simulink model "truckParallelParking"  (R2023a)
settings: Solver=VariableStepAuto  StartTime=0.0  StopTime=30  RelTol=1e-3
values from neighbouring files (symbols this model uses):
  Duration = 30    [ParallelParkingOfTruckTrailerUsingMultistageNonlinearMPC1.m]
  initialPose1 = [-15,-30,pi/2,0]'    [ParallelParkingOfTruckTrailerUsingMultistageNonlinearMPC1.m]
  mdlParas = [truckDimensions.M1;truckDimensions.L1;truckDimensions.L2;             truckDimensions.W1;truckDimensions.W2]    [ParallelParkingOfTruckTrailerUsingMultistageNonlinearMPC1.m]
  numParas = numel(mdlParas) + numel(obsParas)    [ParallelParkingOfTruckTrailerUsingMultistageNonlinearMPC1.m]
  obsParas = [wallLength;wallWidth]    [ParallelParkingOfTruckTrailerUsingMultistageNonlinearMPC1.m]
  pPlanning = planner.horizon    [ParallelParkingOfTruckTrailerUsingMultistageNonlinearMPC1.m]    (also in mpcGeneratePlanner.m = 20)
  pTracking = controller.horizon    [ParallelParkingOfTruckTrailerUsingMultistageNonlinearMPC1.m]
  targetPose2 = [-8,-8,pi/2,0]'    [ParallelParkingOfTruckTrailerUsingMultistageNonlinearMPC1.m]
  tmax = tmin + Tsplan    [ParallelParkingOfTruckTrailerUsingMultistageNonlinearMPC1.m]
  tmin = 2.5    [ParallelParkingOfTruckTrailerUsingMultistageNonlinearMPC1.m]
  Ts = controller.sampleTime    [ParallelParkingOfTruckTrailerUsingMultistageNonlinearMPC1.m]    (also in mpcGeneratePlanner.m = 1)
libraries: mpclib x2, simulink x1
settings Model: Creator=The MathWorks, Inc.  LastModifiedBy=The MathWorks, Inc.
settings SolverCC: MaxZcPerStep=1
settings DebuggingCC: UnconnectedInputMsg=warning  UnconnectedOutputMsg=warning  UnconnectedLineMsg=warning
settings ModelReferenceCC: EnableRefExpFcnMdlSchedulingChecks=on
settings RTWCC: DLArmComputeVersion=19.05

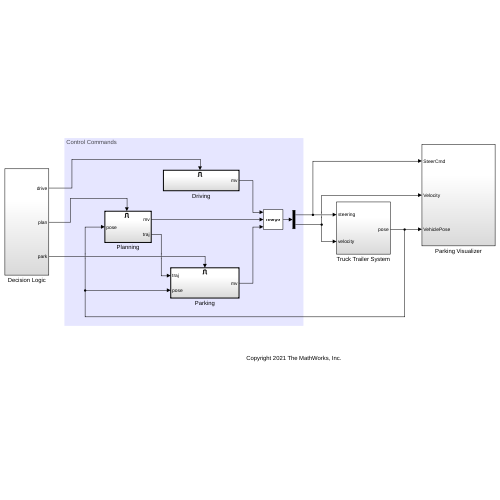
[thumbnail: Simulink's stored preview of the top-level diagram]
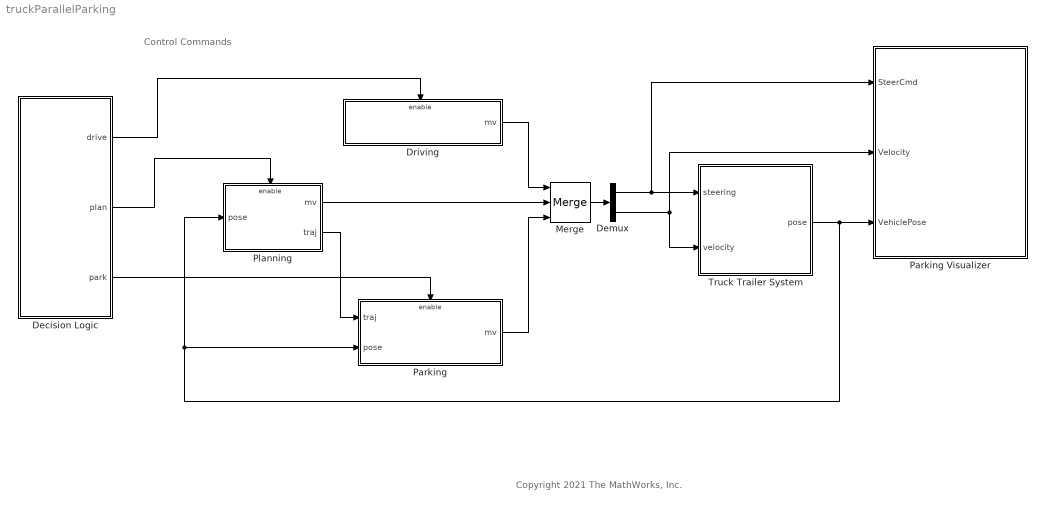
== system truckParallelParking ==
  note: Control Commands
  note: Copyright 2021 The MathWorks, Inc.
  Decision Logic : Subsystem
  Demux : Demux  Outputs=2
  Driving : Subsystem  TreatAsAtomicUnit=on
  Merge : Merge  Inputs=3
  Parking : Subsystem  TreatAsAtomicUnit=on
  Parking Visualizer : Subsystem
  Planning : Subsystem  TreatAsAtomicUnit=on
  Truck Trailer System : Subsystem
  wires:
  Decision Logic/3(park) -> Parking/Enable
  Decision Logic/1(drive) -> Driving/Enable
  Decision Logic/2(plan) -> Planning/Enable
  Merge/1 -> Demux/1
  Driving/1(mv) -> Merge/1
  Demux/1 -> Truck Trailer System/1(steering), Parking Visualizer/1(SteerCmd)
  Demux/2 -> Truck Trailer System/2(velocity), Parking Visualizer/2(Velocity)
  Truck Trailer System/1(pose) -> Parking/2(pose), Planning/1(pose), Parking Visualizer/3(VehiclePose)
  Planning/1(mv) -> Merge/2
  Parking/1(mv) -> Merge/3
  Planning/2(traj) -> Parking/1(traj)

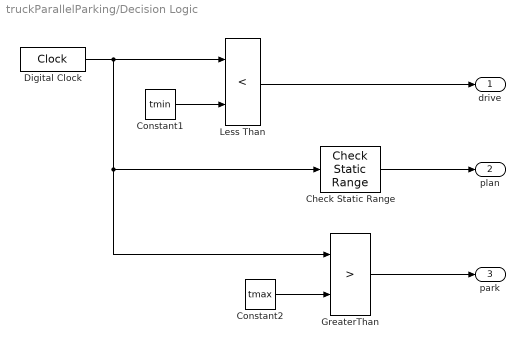
== system truckParallelParking/Decision Logic ==
  Check Static Range : simulink/Model Verification/Check  Static Range  Description=tmin <= u <= tmax  max=tmax  max_included=on  min=tmin  min_included=on  enabled=off  stopWhenAssertionFail=off  export=on  icon=graphic
  Constant1 : Constant  Value=tmin
  Constant2 : Constant  Value=tmax
  Digital Clock : DigitalClock  SampleTime=0.1
  GreaterThan : RelationalOperator  Operator=>  OutDataTypeStr=boolean  RndMeth=Simplest  InputSameDT=off
  Less Than : RelationalOperator  Operator=<  OutDataTypeStr=boolean  RndMeth=Simplest  InputSameDT=off
  drive : Outport
  plan : Outport  Port=2
  park : Outport  Port=3
  wires:
  Constant1/1 -> Less Than/2
  Less Than/1 -> drive/1
  Digital Clock/1 -> GreaterThan/1, Check Static Range/1, Less Than/1
  Check Static Range/1 -> plan/1
  Constant2/1 -> GreaterThan/2
  GreaterThan/1 -> park/1

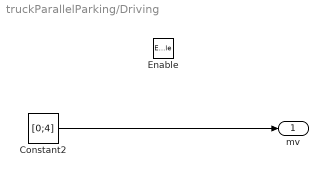
== system truckParallelParking/Driving ==
  Enable : EnablePort  StatesWhenEnabling=reset
  Constant2 : Constant  Value=[0;4]  VectorParams1D=off
  mv : Outport
  wires:
  Constant2/1 -> mv/1

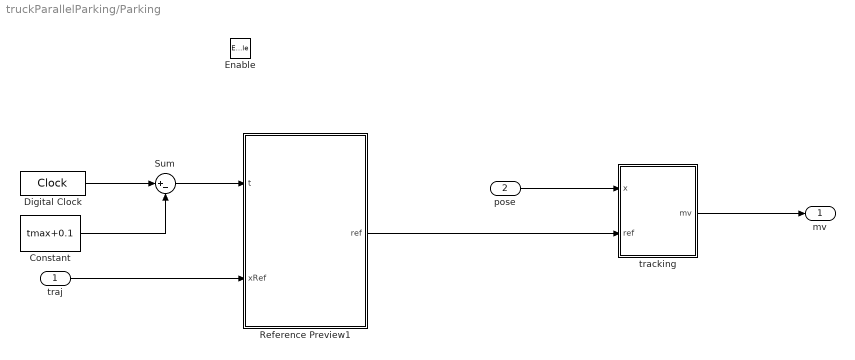
== system truckParallelParking/Parking ==
  traj : Inport
  pose : Inport  Port=2
  Enable : EnablePort  StatesWhenEnabling=reset
  Constant : Constant  Value=tmax+0.1
  Digital Clock : DigitalClock  SampleTime=0.1
  Reference Preview1 : MATLAB Function  TreatAsAtomicUnit=on
  Sum : Sum  Inputs=|+-
  tracking : Subsystem
  mv : Outport
  wires:
  traj/1 -> Reference Preview1/2(xRef)
  Reference Preview1/1(ref) -> tracking/2(ref)
  pose/1 -> tracking/1(x)
  tracking/1(mv) -> mv/1
  Sum/1 -> Reference Preview1/1(t)
  Digital Clock/1 -> Sum/1
  Constant/1 -> Sum/2

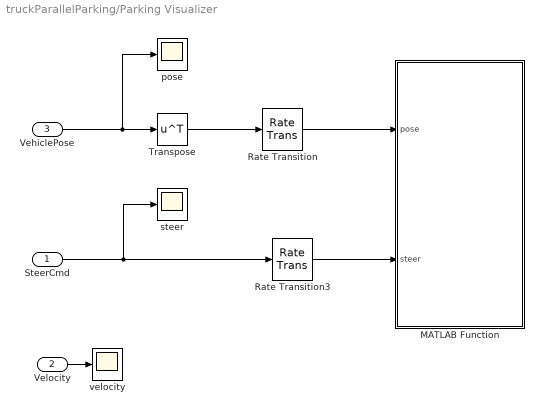
== system truckParallelParking/Parking Visualizer ==
  SteerCmd : Inport
  Velocity : Inport  Port=2
  VehiclePose : Inport  Port=3
  MATLAB Function : MATLAB Function  TreatAsAtomicUnit=on
  Rate Transition : RateTransition  OutPortSampleTime=0.1
  Rate Transition3 : RateTransition  OutPortSampleTime=0.1
  Transpose : Math  Operator=transpose
  pose : Scope
  steer : Scope
  velocity : Scope
  wires:
  Rate Transition/1 -> MATLAB Function/1(pose)
  VehiclePose/1 -> pose/1, Transpose/1
  Rate Transition3/1 -> MATLAB Function/2(steer)
  SteerCmd/1 -> steer/1, Rate Transition3/1
  Transpose/1 -> Rate Transition/1
  Velocity/1 -> velocity/1

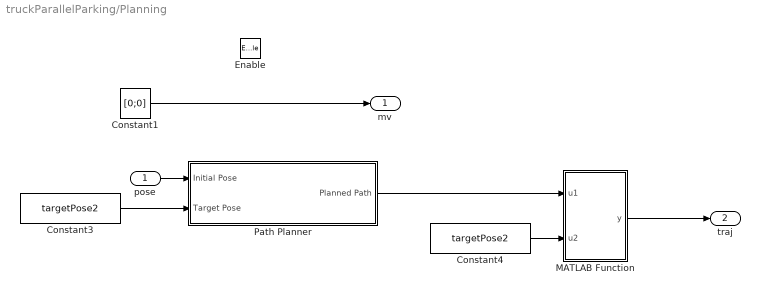
== system truckParallelParking/Planning ==
  pose : Inport
  Enable : EnablePort  StatesWhenEnabling=reset
  Constant1 : Constant  Value=[0;0]  VectorParams1D=off
  Constant3 : Constant  Value=targetPose2
  Constant4 : Constant  Value=targetPose2
  MATLAB Function : MATLAB Function  TreatAsAtomicUnit=on
  Path Planner : Subsystem
  mv : Outport
  traj : Outport  Port=2
  wires:
  Constant1/1 -> mv/1
  Constant3/1 -> Path Planner/2(Target Pose)
  pose/1 -> Path Planner/1(Initial Pose)
  MATLAB Function/1(y) -> traj/1
  Constant4/1 -> MATLAB Function/2(u2)
  Path Planner/1(Planned Path) -> MATLAB Function/1(u1)

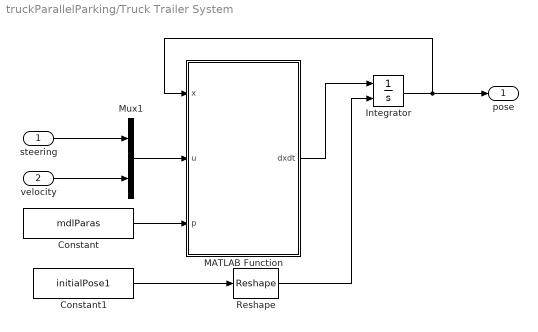
== system truckParallelParking/Truck Trailer System ==
  steering : Inport
  velocity : Inport  Port=2
  Constant : Constant  Value=mdlParas
  Constant1 : Constant  Value=initialPose1
  Integrator : Integrator  InitialConditionSource=external
  MATLAB Function : MATLAB Function  TreatAsAtomicUnit=on
  Mux1 : Mux  Inputs=2
  Reshape : Reshape  OutputDimensionality=Customize  OutputDimensions=[4,1]
  pose : Outport
  wires:
  MATLAB Function/1(dxdt) -> Integrator/1
  Constant1/1 -> Reshape/1
  Integrator/1 -> pose/1, MATLAB Function/1(x)
  velocity/1 -> Mux1/2
  Reshape/1 -> Integrator/2
  Mux1/1 -> MATLAB Function/2(u)
  steering/1 -> Mux1/1
  Constant/1 -> MATLAB Function/3(p)

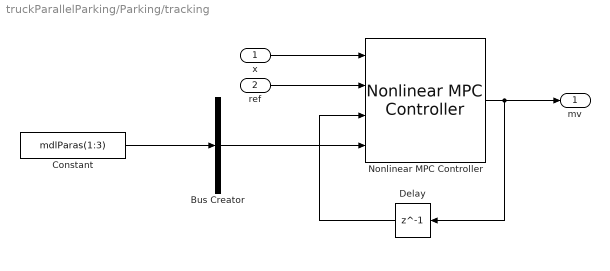
== system truckParallelParking/Parking/tracking ==
  x : Inport
  ref : Inport  Port=2
  Bus Creator : BusCreator  Inputs=1  OutDataTypeStr=Bus: parasBusObject  NonVirtualBus=on
      settings: InheritFromInputs=off
  Constant : Constant  Value=mdlParas(1:3)
  Delay : Delay  DelayLength=1
  Nonlinear MPC Controller : mpclib/Nonlinear MPC Controller  SCDEnableBlockLinearizationSpecification=on  nlmpcobj=trackingObj  UseObjectTs=on  UseMEX=off  md_enabled=off  mvtarget_enabled=off  param_enabled=on  cost_enabled=off  mvseq_enabled=off  stateseq_enabled=off  ovseq_enabled=off  slack_enabled=off  status_enabled=off  ov_min=off  ov_max=off  mv_min=off  mv_max=off  mvrate_min=off  mvrate_max=off  state_min=off  state_max=off  ov_weight=off  mv_weight=off  mvrate_weight=off  ecr_weight=off  nlp_initialize=off
  mv : Outport
  wires:
  ref/1 -> Nonlinear MPC Controller/2
  Nonlinear MPC Controller/1 -> mv/1, Delay/1
  Delay/1 -> Nonlinear MPC Controller/3
  x/1 -> Nonlinear MPC Controller/1
  Bus Creator/1 -> Nonlinear MPC Controller/4
  Constant/1 -> Bus Creator/1

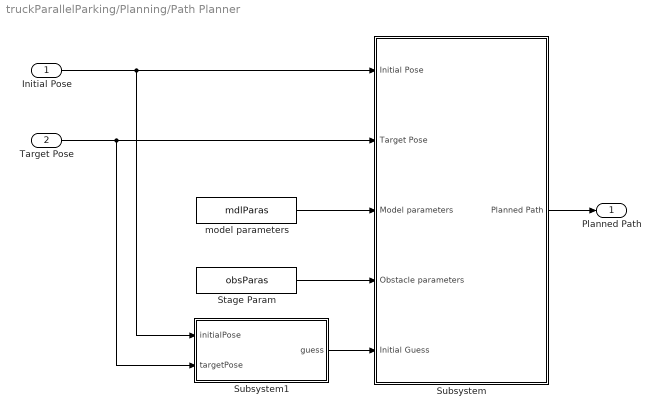
== system truckParallelParking/Planning/Path Planner ==
  Initial Pose : Inport
  Target Pose : Inport  Port=2
  Stage Param : Constant  Value=obsParas  VectorParams1D=off
  Subsystem : Subsystem
  Subsystem1 : Subsystem
  model parameters : Constant  Value=mdlParas  VectorParams1D=off
  Planned Path : Outport
  wires:
  Target Pose/1 -> Subsystem1/2(targetPose), Subsystem/2(Target Pose)
  Stage Param/1 -> Subsystem/4(Obstacle parameters)
  Initial Pose/1 -> Subsystem1/1(initialPose), Subsystem/1(Initial Pose)
  model parameters/1 -> Subsystem/3(Model parameters)
  Subsystem/1(Planned Path) -> Planned Path/1
  Subsystem1/1(guess) -> Subsystem/5(Initial Guess)

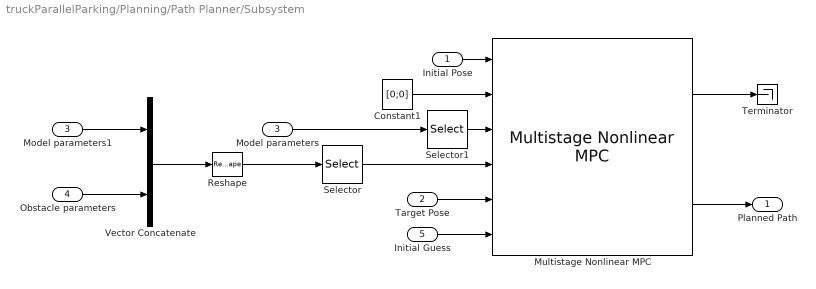
== system truckParallelParking/Planning/Path Planner/Subsystem ==
  Initial Pose : Inport
  Target Pose : Inport  Port=2
  Model parameters : Inport  Port=3
  Obstacle parameters : Inport  Port=4
  Initial Guess : Inport  Port=5
  Constant1 : Constant  Value=[0;0]
  Model parameters1 : InportShadow  Port=3
  Multistage Nonlinear MPC : mpclib/Multistage Nonlinear MPC  SCDEnableBlockLinearizationSpecification=on  nlmpcobj=planningObj  UseObjectTs=on  TsControl=2  UseMEX=off  md_enabled=off  stateparam_enabled=on  stageparam_enabled=on  cost_enabled=off  mvseq_enabled=off  stateseq_enabled=on  slack_enabled=off  status_enabled=off  mv_min=off  mv_max=off  mvrate_min=off  mvrate_max=off  state_min=off  state_max=off  terminal_state=on  nlp_initialize=on
  Reshape : Reshape  OutputDimensionality=Customize  OutputDimensions=[1,numParas]
  Selector : Selector  NumberOfDimensions=2  InputPortWidth=3  IndexOptions=Select all,Index vector (dialog)  Indices=[1 3],repmat([1:numParas]',pPlanning,1)  OutputSizes=1,1
  Selector1 : Selector  InputPortWidth=5  IndexOptions=Index vector (dialog)  Indices=[1 2 3]  OutputSizes=1
  Terminator : Terminator
  Vector Concatenate : Concatenate
  Planned Path : Outport
  wires:
  Target Pose/1 -> Multistage Nonlinear MPC/5
  Initial Pose/1 -> Multistage Nonlinear MPC/1
  Constant1/1 -> Multistage Nonlinear MPC/2
  Selector/1 -> Multistage Nonlinear MPC/4
  Multistage Nonlinear MPC/2 -> Planned Path/1
  Multistage Nonlinear MPC/1 -> Terminator/1
  Model parameters/1 -> Selector1/1
  Initial Guess/1 -> Multistage Nonlinear MPC/6
  Vector Concatenate/1 -> Reshape/1
  Model parameters1/1 -> Vector Concatenate/1
  Obstacle parameters/1 -> Vector Concatenate/2
  Reshape/1 -> Selector/1
  Selector1/1 -> Multistage Nonlinear MPC/3

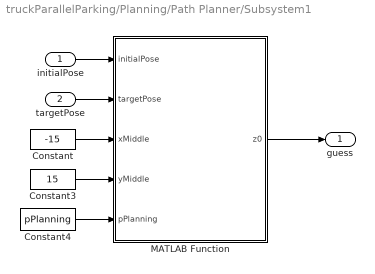
== system truckParallelParking/Planning/Path Planner/Subsystem1 ==
  initialPose : Inport
  targetPose : Inport  Port=2
  Constant : Constant  Value=-15
  Constant3 : Constant  Value=15
  Constant4 : Constant  Value=pPlanning
  MATLAB Function : MATLAB Function  TreatAsAtomicUnit=on
  guess : Outport
  wires:
  MATLAB Function/1(z0) -> guess/1
  Constant/1 -> MATLAB Function/3(xMiddle)
  Constant3/1 -> MATLAB Function/4(yMiddle)
  Constant4/1 -> MATLAB Function/5(pPlanning)
  initialPose/1 -> MATLAB Function/1(initialPose)
  targetPose/1 -> MATLAB Function/2(targetPose)

== matlab function truckParallelParking/Planning/Path Planner/Subsystem1/MATLAB Function ==
  data: initialPose input; z0 output; targetPose input; xMiddle input; yMiddle input; pPlanning input
function z0 = fcn(initialPose,targetPose,xMiddle,yMiddle,pPlanning)

[z0,~,~] = mpcGenerateInitialGuess(initialPose,targetPose,xMiddle,yMiddle,pPlanning);

== matlab function truckParallelParking/Truck Trailer System/MATLAB Function ==
  settings: updateMethod=DISCRETE  sampleTime=0.1
  data: x input; u input; dxdt output; p input
function dxdt = fcn(x, u,p)%#codegen
dxdt = zeros(4,1);
dxdt = stateFcnTruck(x, u, p);

== matlab function truckParallelParking/Parking Visualizer/MATLAB Function ==
  data: pose input; steer input; truckDimensions parameter
function visualizeParkingValet(pose, steer, truckDimensions)

%visualizePath Display simulation results.

coder.extrinsic('helperSLVisualizeParkingTruck');

helperSLVisualizeParkingTruck(pose, steer, truckDimensions)

== matlab function truckParallelParking/Parking/Reference Preview1 ==
  data: t input; ref output; xRef input; Ts parameter size=[1,1]; pTracking parameter size=[1,1]; Duration parameter size=[1,1]
function ref = fcn(t,xRef, Ts, pTracking, Duration)
Tend = Duration;
T = t+(1:pTracking)*Ts;
T = min(T,Tend);
time = Ts*(1:length(xRef));
ref = interp1(time,xRef,T);

== matlab function truckParallelParking/Planning/MATLAB Function ==
  data: u1 input; y output; u2 input
function y = fcn(u1,u2)

traj = mpcInterpolatePathSL(u1,u2);
Ts = 0.1;
Duration = 30;
Tsteps = Duration/Ts;
y = [traj;repmat(traj(end,:),Tsteps-size(traj,1),1)];
